simulink model "verySimpleSystem"  (R2023a)
settings: Solver=VariableStepAuto  StartTime=0.0  StopTime=0.1  RelTol=1e-3
InitFcn:
  | initTest
values from neighbouring files (symbols this model uses):
  modulationFrequency = 40e3    (= 40000)    [initTest.m]
  RFCarrier = 1e6    (= 1000000)    [initTest.m]
libraries: simrfV2util1 x3, simrfV2sources1 x2, simrfV2elements x2, simrfV2_lib x1
settings Model: Creator=Hossein  LastModifiedBy=Hossein

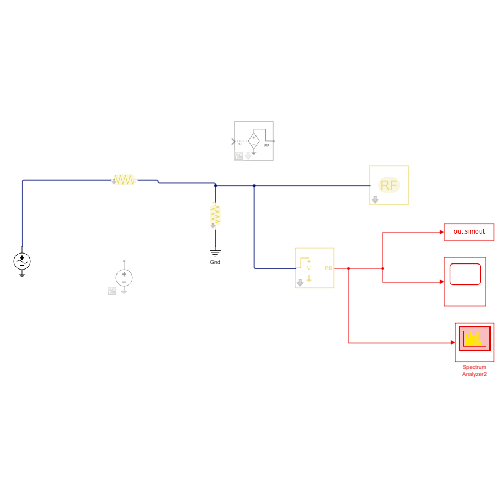
[thumbnail: Simulink's stored preview of the top-level diagram]
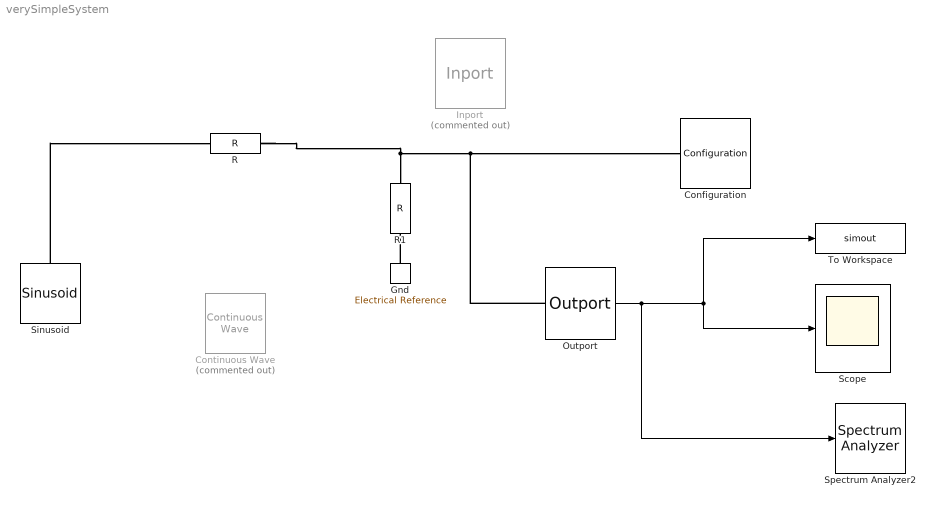
== system verySimpleSystem ==
  Configuration : simrfV2util1/Configuration  AutoFreq=off  Tones=[modulationFrequency, RFCarrier] Hz  Harmonics=[7]  NormalizeCarrierPower=on  SolverType=Auto  UseCCode=on  StepSize=1/(RFCarrier*10) s  AddNoise=on  defaultRNG=on  Seed=0  Temperature=290.0 K  SolverDelFlag=0  AbsTol=1e-6  RelTol=1e-3  MaxIter=10  ErrorEstimationType=2-norm over all variables  EnableInterpFilter=on  HiddenFIRfilterControllerParam=off  SmallSignalApprox=off  AllSimFreqs=on  SimFreqs=[] Hz  SimFreqsInternal=[]  SamplesPerFrame=1
  Continuous Wave : simrfV2sources1/Continuous Wave  Commented=on  CWSourceType=Ideal voltage  Z0=0  IVoltage=1 V  ICurrent=0 A  MagPower=0 W  QVoltage=0 V  QCurrent=0 A  AnglePower=0  CarrierFreq=1 MHz  AddPhaseNoise=off  PhaseNoiseOffset=1  PhaseNoiseLevel=-Inf  AutoImpulseLength=on  ImpulseLength=1e-10 s  InternalGrounding=on
  Gnd : simrfV2_lib/Elements/Electrical Reference
      settings: LibrarySourceBlock=simrfV2elements/Gnd  InternalSimscapePortConfiguration="{\"Bottom\":[],\"Left\":[{\"id\":\"V\",\"label\":\"\",\"type\":\"foundation.rf.circuitenvelope\"}],\"Right\":[],\"Top\":[]}"
  Inport : simrfV2util1/Inport  Commented=on  SimulinkInputSignalType=Ideal voltage  CarrierFreq=0 Hz  ZS=0  UseSqWave=off  NumCoeff=10  Bias=0  DutyCyc=50  InternalGrounding=on
  Outport : simrfV2util1/Outport  SensorType=Ideal voltage  OutputFormat=Real Passband  CarrierFreq=RFCarrier Hz  ZL=Inf  InternalGrounding=on  StepSize=1.25e-07 s  AutoStep=on  HalfPolyphaseLength=24
  R : simrfV2elements/R  classname=resistor  Resistance=1 Ohm  AddNoise=on
  R1 : simrfV2elements/R  classname=resistor  Resistance=1 Ohm  AddNoise=on
  Scope : Scope
  Sinusoid : simrfV2sources1/Sinusoid  SineSourceType=Ideal voltage  VO_I=0 V  IO_I=0 A  VO_Q=0 V  IO_Q=0 A  VA_I=modulationAmplitude V  IA_I=0 A  VA_Q=0 V  IA_Q=0 A  Fmod=modulationFrequency Hz  TD=0 s  CarrierFreq=RFCarrier Hz  InternalGrounding=on
  Spectrum Analyzer2 : SpectrumAnalyzer  Tag=simrfV2util1/Spectrum Analyzer  WindowPosition=[560.000000,290.000000,800.000000,500.000000,]  Visible=on  ScopeFrameLocation=window  Span=10000000  StartFrequency=-5000000  StopFrequency=5000000  YLimits=[-153.92745851,33.48812322]  ExpandToolstrip=on
  To Workspace : ToWorkspace  VariableName=simout  SampleTime=-1
      settings: Save2DSignal=2-D array (concatenate along first dimension)
  wires:
  Outport/1 -> Spectrum Analyzer2/1, To Workspace/1, Scope/1
  connections:
  Gnd/LConn1 -- R1/RConn1
  R/RConn1 -- Outport/LConn1 -- Configuration/LConn1 -- R1/LConn1
  Sinusoid/LConn1 -- R/LConn1
